simulink model "sampleModel2008"  (R2023a)
settings: Solver=VariableStepAuto  StartTime=0.0  StopTime=10.0  RelTol=1e-3
libraries: hdlsllib x5, simulink x1
settings Model: Creator=user1  LastModifiedBy=user1

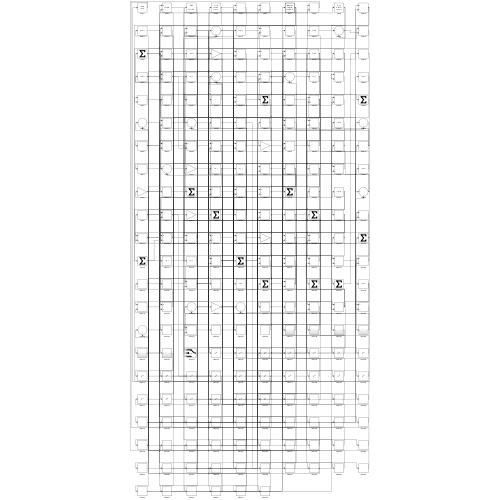
[thumbnail: Simulink's stored preview of the top-level diagram]
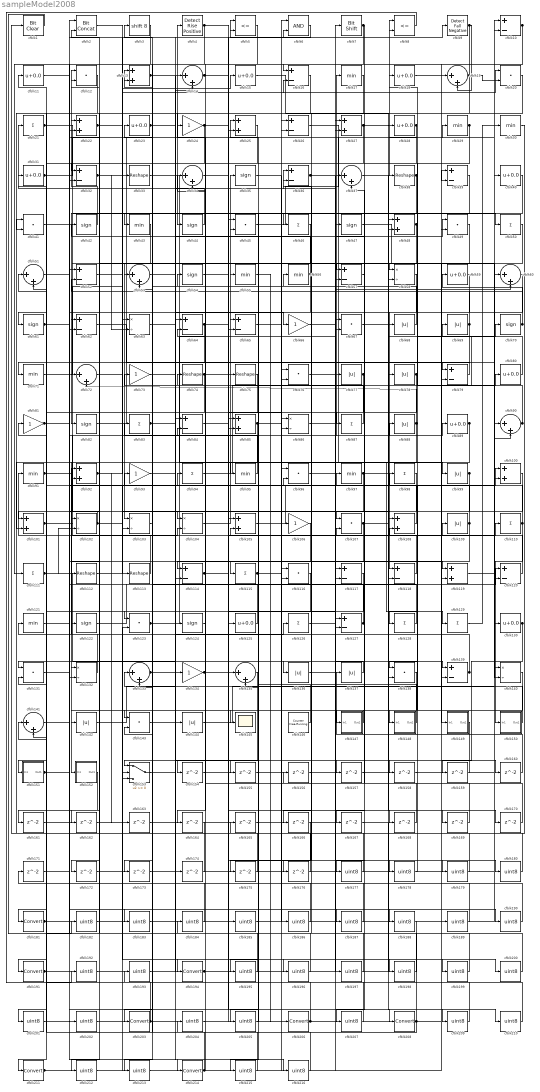
== system sampleModel2008 ==
  cfblk1 : simulink/Logic and Bit Operations/Bit Clear  iBit=0
      settings: LibrarySourceBlock=|
      | hdlsllib/Logic and Bit
      | Operations/Bit Clear
  cfblk{10,16,26,32,36,39,52,57,62,64..65,79,84,114,117..118,120,127,139} (19 alike) : Sum  Inputs=+-
  cfblk{13,22,25,27,48,85,92,100..101,105,108,119} (12 alike) : Sum
  cfblk{58,63,86,102..104,132,140} (8 alike) : Product  Inputs=*/  RndMeth=Zero  SaturateOnIntegerOverflow=on
  cfblk{24,66,73,81,93,106,134} (7 alike) : Gain
  cfblk{12,20,41,45,49,67,76,96,107,116,123,131,138,143} (14 alike) : DotProduct  OutDataTypeStr=Inherit: Inherit via internal rule
  cfblk{68..69,77..78,88,99,109,136..137,142,144} (11 alike) : Abs  SaturateOnIntegerOverflow=off
  cfblk{11,15,18,23,28,31,40,59,80,89,125,130} (12 alike) : Bias  Bias=0.0  SaturateOnIntegerOverflow=off
  cfblk{21,46,50,83,87,94,98,110..111,115,126,128..129} (13 alike) : Sum  Inputs=+
  cfblk{33,38,74..75,112..113} (6 alike) : Reshape
  cfblk{17,29..30,43,55..56,71,91,95,97,121} (11 alike) : MinMax
  cfblk{35,42,44,47,54,61,70,82,122,124} (10 alike) : Signum
  cfblk{14,19,34,37,51,53,60,72,90,133,135,141} (12 alike) : Sum  Inputs=|++
  cfblk145 : Scope
  cfblk146 : hdlsllib/Sources/Counter Free-Running  NumBits=16  tsamp=-1
  cfblk147 : Subsystem
      settings: LibrarySourceBlock=|
      | hdlsllib/Ports &
      | Subsystems/Subsystem
  cfblk148 : Subsystem
      settings: LibrarySourceBlock=|
      | hdlsllib/Ports &
      | Subsystems/Subsystem
  cfblk149 : Subsystem
      settings: LibrarySourceBlock=|
      | hdlsllib/Ports &
      | Subsystems/Subsystem
  cfblk150 : Subsystem
      settings: LibrarySourceBlock=|
      | hdlsllib/Ports &
      | Subsystems/Subsystem
  cfblk151 : Subsystem
      settings: LibrarySourceBlock=|
      | hdlsllib/Ports &
      | Subsystems/Subsystem
  cfblk152 : Subsystem
      settings: LibrarySourceBlock=|
      | hdlsllib/Ports &
      | Subsystems/Subsystem
  cfblk153 : Switch  SaturateOnIntegerOverflow=off  InputSameDT=off
  cfblk{154..176} (23 alike) : Delay  SampleTime=1
  cfblk{177..180,182..190,192..193,195..202,204..205,207,209..210,212..213,215..216} (32 alike) : DataTypeConversion  OutDataTypeStr=uint8  SaturateOnIntegerOverflow=off  RndMeth=Floor
  cfblk{181,191,194,203,206,208,211,214} (8 alike) : DataTypeConversion  SaturateOnIntegerOverflow=off  RndMeth=Floor
  cfblk2 : hdlsllib/Logic and Bit Operations/Bit Concat  numInputs=2
  cfblk3 : ArithShift  BitShiftNumber=8
  cfblk4 : hdlsllib/Logic and Bit Operations/Detect Rise Positive  vinit=0  OutDataTypeStr=boolean
  cfblk5 : RelationalOperator  Operator=<=  OutDataTypeStr=boolean  InputSameDT=off
  cfblk6 : Logic  AllPortsSameDT=off  OutDataTypeStr=boolean
  cfblk7 : hdlsllib/Logic and Bit Operations/Bit Shift  mode=Shift Left Logical  N=0
  cfblk8 : RelationalOperator  Operator=<=  OutDataTypeStr=boolean  InputSameDT=off
  cfblk9 : hdlsllib/Logic and Bit Operations/Detect Fall Negative  vinit=0  OutDataTypeStr=boolean
  wires:
  cfblk42/1 -> cfblk12/1
  cfblk129/1 -> cfblk30/1
  cfblk58/1 -> cfblk118/1
  cfblk33/1 -> cfblk129/1
  cfblk3/1 -> cfblk111/1
  cfblk104/1 -> cfblk35/1
  cfblk51/1 -> cfblk214/1
  cfblk41/1 -> cfblk108/1
  cfblk17/1 -> cfblk44/1
  cfblk48/1 -> cfblk58/1, cfblk102/1, cfblk213/1
  cfblk47/1 -> cfblk149/1(In1)
  cfblk39/1 -> cfblk82/1
  cfblk123/1 -> cfblk65/1, cfblk187/1, cfblk216/1
  cfblk118/1 -> cfblk91/1
  cfblk91/1 -> cfblk17/1, cfblk88/1
  cfblk89/1 -> cfblk152/1(In1), cfblk138/1
  cfblk26/1 -> cfblk99/1
  cfblk4/1 -> cfblk133/2, cfblk180/1
  cfblk107/1 -> cfblk114/1, cfblk169/1
  cfblk22/1 -> cfblk132/1, cfblk16/2
  cfblk7/1 -> cfblk87/1, cfblk25/2, cfblk32/2
  cfblk69/1 -> cfblk52/2, cfblk201/1
  cfblk49/1 -> cfblk68/1
  cfblk149/1(Out1) -> cfblk137/1
  cfblk94/1 -> cfblk7/1
  cfblk148/1(Out1) -> cfblk56/1
  cfblk108/1 -> cfblk11/1
  cfblk109/1 -> cfblk13/2, cfblk176/1
  cfblk82/1 -> cfblk4/1
  cfblk50/1 -> cfblk103/1
  cfblk43/1 -> cfblk53/1
  cfblk32/1 -> cfblk113/1, cfblk63/2
  cfblk103/1 -> cfblk53/2
  cfblk85/1 -> cfblk101/2, cfblk160/1
  cfblk9/1 -> cfblk19/2, cfblk164/1
  cfblk110/1 -> cfblk150/1(In1), cfblk47/1
  cfblk141/1 -> cfblk208/1
  cfblk11/1 -> cfblk115/1
  cfblk115/1 -> cfblk26/1, cfblk109/1
  cfblk101/1 -> cfblk89/1, cfblk104/2
  cfblk73/1 -> cfblk134/1
  cfblk127/1 -> cfblk94/1, cfblk122/1
  cfblk70/1 -> cfblk59/1, cfblk37/2
  cfblk132/1 -> cfblk81/1
  cfblk55/1 -> cfblk206/1
  cfblk14/1 -> cfblk170/1, cfblk198/1
  cfblk88/1 -> cfblk147/1(In1), cfblk72/2, cfblk151/1(In1)
  cfblk71/1 -> cfblk33/1
  cfblk28/1 -> cfblk65/2, cfblk46/1
  cfblk6/1 -> cfblk5/1
  cfblk139/1 -> cfblk92/1, cfblk77/1, cfblk25/1
  cfblk144/1 -> cfblk10/1
  cfblk16/1 -> cfblk62/1
  cfblk44/1 -> cfblk21/1
  cfblk81/1 -> cfblk62/2, cfblk107/1
  cfblk99/1 -> cfblk153/2, cfblk195/1
  cfblk78/1 -> cfblk103/2, cfblk215/1
  cfblk37/1 -> cfblk8/1
  cfblk150/1(Out1) -> cfblk133/1
  cfblk19/1 -> cfblk71/1, cfblk16/1, cfblk20/2
  cfblk40/1 -> cfblk128/1
  cfblk10/1 -> cfblk39/2, cfblk22/2
  cfblk146/1 -> cfblk54/1
  cfblk60/1 -> cfblk142/1
  cfblk80/1 -> cfblk18/1
  cfblk130/1 -> cfblk140/2, cfblk159/1
  cfblk2/1 -> cfblk194/1
  cfblk64/1 -> cfblk127/2, cfblk212/1
  cfblk23/1 -> cfblk8/2, cfblk66/1
  cfblk113/1 -> cfblk22/1
  cfblk116/1 -> cfblk191/1
  cfblk95/1 -> cfblk83/1
  cfblk92/1 -> cfblk9/1, cfblk163/1
  cfblk111/1 -> cfblk144/1, cfblk102/2
  cfblk93/1 -> cfblk49/1
  cfblk29/1 -> cfblk148/1(In1), cfblk32/1
  cfblk135/1 -> cfblk203/1
  cfblk142/1 -> cfblk64/1
  cfblk67/1 -> cfblk38/1
  cfblk68/1 -> cfblk13/1
  cfblk128/1 -> cfblk36/1
  cfblk87/1 -> cfblk73/1
  cfblk61/1 -> cfblk29/1, cfblk190/1
  cfblk112/1 -> cfblk100/1
  cfblk75/1 -> cfblk181/1
  cfblk134/1 -> cfblk20/1, cfblk6/2, cfblk210/1
  cfblk18/1 -> cfblk19/1
  cfblk131/1 -> cfblk100/2
  cfblk97/1 -> cfblk70/1, cfblk153/1
  cfblk21/1 -> cfblk57/1, cfblk50/1
  cfblk137/1 -> cfblk131/1
  cfblk13/1 -> cfblk79/1, cfblk119/2
  cfblk38/1 -> cfblk95/1, cfblk153/3
  cfblk15/1 -> cfblk78/1
  cfblk90/1 -> cfblk28/1, cfblk69/1
  cfblk79/1 -> cfblk72/1
  cfblk147/1(Out1) -> cfblk145/1
  cfblk117/1 -> cfblk211/1
  cfblk66/1 -> cfblk67/1
  cfblk31/1 -> cfblk90/1, cfblk6/1
  cfblk151/1(Out1) -> cfblk120/1, cfblk5/2
  cfblk133/1 -> cfblk126/1, cfblk157/1
  cfblk63/1 -> cfblk124/1
  cfblk122/1 -> cfblk85/1
  cfblk45/1 -> cfblk10/2
  cfblk119/1 -> cfblk140/1
  cfblk86/1 -> cfblk60/2
  cfblk74/1 -> cfblk123/1, cfblk67/2
  cfblk52/1 -> cfblk15/1
  cfblk143/1 -> cfblk37/1
  cfblk56/1 -> cfblk42/1, cfblk132/2
  cfblk12/1 -> cfblk41/2
  cfblk120/1 -> cfblk92/2
  cfblk72/1 -> cfblk63/1
  cfblk114/1 -> cfblk85/2, cfblk119/1, cfblk110/1, cfblk168/1
  cfblk77/1 -> cfblk136/1, cfblk104/1
  cfblk102/1 -> cfblk97/1, cfblk101/1
  cfblk153/1 -> cfblk14/2
  cfblk105/1 -> cfblk48/2
  cfblk24/1 -> cfblk105/1, cfblk43/1
  cfblk5/1 -> cfblk143/1
  cfblk62/1 -> cfblk130/1
  cfblk125/1 -> cfblk3/1
  cfblk83/1 -> cfblk36/2, cfblk173/1
  cfblk27/1 -> cfblk61/1, cfblk139/2
  cfblk46/1 -> cfblk112/1
  cfblk36/1 -> cfblk139/1, cfblk199/1
  cfblk59/1 -> cfblk79/2
  cfblk54/1 -> cfblk86/2
  cfblk136/1 -> cfblk80/1
  cfblk124/1 -> cfblk154/1
  cfblk154/1 -> cfblk118/2
  cfblk140/1 -> cfblk155/1
  cfblk155/1 -> cfblk48/1
  cfblk157/1 -> cfblk60/1
  cfblk126/1 -> cfblk158/1
  cfblk158/1 -> cfblk39/1
  cfblk159/1 -> cfblk127/1
  cfblk160/1 -> cfblk108/2
  cfblk152/1(Out1) -> cfblk161/1
  cfblk161/1 -> cfblk114/2
  cfblk138/1 -> cfblk162/1
  cfblk162/1 -> cfblk26/2
  cfblk164/1 -> cfblk1/1
  cfblk30/1 -> cfblk165/1
  cfblk165/1 -> cfblk57/2
  cfblk20/1 -> cfblk166/1
  cfblk100/1 -> cfblk167/1
  cfblk168/1 -> cfblk107/2
  cfblk169/1 -> cfblk105/2
  cfblk170/1 -> cfblk64/2
  cfblk25/1 -> cfblk172/1
  cfblk172/1 -> cfblk90/2
  cfblk173/1 -> cfblk58/2
  cfblk53/1 -> cfblk174/1
  cfblk174/1 -> cfblk52/1
  cfblk106/1 -> cfblk175/1
  cfblk175/1 -> cfblk41/1
  cfblk176/1 -> cfblk12/2
  cfblk98/1 -> cfblk177/1
  cfblk177/1 -> cfblk45/2
  cfblk65/1 -> cfblk178/1
  cfblk178/1 -> cfblk98/1
  cfblk156/1 -> cfblk179/1
  cfblk179/1 -> cfblk45/1
  cfblk180/1 -> cfblk156/1
  cfblk181/1 -> cfblk27/2, cfblk40/1, cfblk27/1
  cfblk1/1 -> cfblk182/1
  cfblk182/1 -> cfblk75/1
  cfblk121/1 -> cfblk183/1
  cfblk183/1 -> cfblk125/1
  cfblk184/1 -> cfblk121/1
  cfblk84/1 -> cfblk185/1
  cfblk185/1 -> cfblk120/2
  cfblk35/1 -> cfblk186/1
  cfblk186/1 -> cfblk84/1
  cfblk187/1 -> cfblk84/2
  cfblk34/1 -> cfblk188/1
  cfblk189/1 -> cfblk34/1
  cfblk190/1 -> cfblk34/2
  cfblk191/1 -> cfblk171/1, cfblk14/1
  cfblk8/1 -> cfblk192/1
  cfblk192/1 -> cfblk116/1
  cfblk188/1 -> cfblk193/1
  cfblk193/1 -> cfblk116/2
  cfblk194/1 -> cfblk138/2, cfblk24/1
  cfblk195/1 -> cfblk2/1
  cfblk163/1 -> cfblk196/1
  cfblk196/1 -> cfblk2/2
  cfblk96/1 -> cfblk197/1
  cfblk197/1 -> cfblk131/2
  cfblk198/1 -> cfblk96/1
  cfblk199/1 -> cfblk96/2
  cfblk76/1 -> cfblk200/1
  cfblk200/1 -> cfblk23/1
  cfblk201/1 -> cfblk76/1
  cfblk171/1 -> cfblk202/1
  cfblk202/1 -> cfblk76/2
  cfblk203/1 -> cfblk31/1, cfblk49/2
  cfblk204/1 -> cfblk135/1
  cfblk166/1 -> cfblk205/1
  cfblk205/1 -> cfblk135/2
  cfblk206/1 -> cfblk93/1, cfblk86/1
  cfblk57/1 -> cfblk207/1
  cfblk207/1 -> cfblk55/1
  cfblk208/1 -> cfblk204/1, cfblk74/1
  cfblk167/1 -> cfblk209/1
  cfblk209/1 -> cfblk141/1
  cfblk210/1 -> cfblk141/2
  cfblk211/1 -> cfblk189/1, cfblk123/2
  cfblk212/1 -> cfblk117/1
  cfblk213/1 -> cfblk117/2
  cfblk214/1 -> cfblk184/1, cfblk143/2, cfblk106/1
  cfblk215/1 -> cfblk51/1
  cfblk216/1 -> cfblk51/2

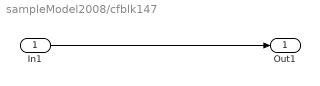
== system sampleModel2008/cfblk147 ==
  In1 : Inport
  Out1 : Outport
  wires:
  In1/1 -> Out1/1

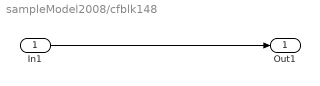
== system sampleModel2008/cfblk148 ==
  In1 : Inport
  Out1 : Outport
  wires:
  In1/1 -> Out1/1

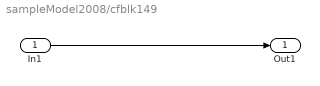
== system sampleModel2008/cfblk149 ==
  In1 : Inport
  Out1 : Outport
  wires:
  In1/1 -> Out1/1

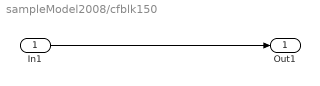
== system sampleModel2008/cfblk150 ==
  In1 : Inport
  Out1 : Outport
  wires:
  In1/1 -> Out1/1

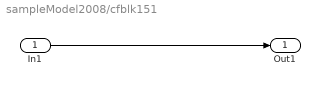
== system sampleModel2008/cfblk151 ==
  In1 : Inport
  Out1 : Outport
  wires:
  In1/1 -> Out1/1

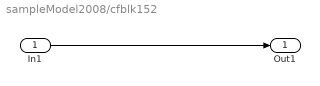
== system sampleModel2008/cfblk152 ==
  In1 : Inport
  Out1 : Outport
  wires:
  In1/1 -> Out1/1
